simulink model "MPCtest"  (R2016a)
settings: Solver=ode45  StartTime=0.0  StopTime=3600  RelTol=1e-3
StartFcn:
  | % clear all
  | load('mpc');
undefined symbols (not defined in the file or in its folder): model_arx, model_bj, model_oe, model_tf
libraries: slident x5, mpclib x1, realtime_pacer_lib x1
settings Model: Creator=johnh  LastModifiedBy=tiago
settings DataIOCC: SaveFormat=StructureWithTime
settings OptimizationCC: BlockReduction=off  DefaultParameterBehavior=Inlined  BufferReuse=off
settings HardwareCC: ProdWordSize=32  ProdHWDeviceType=Specified
settings ConfigComp: CovModelRefEnable=Off

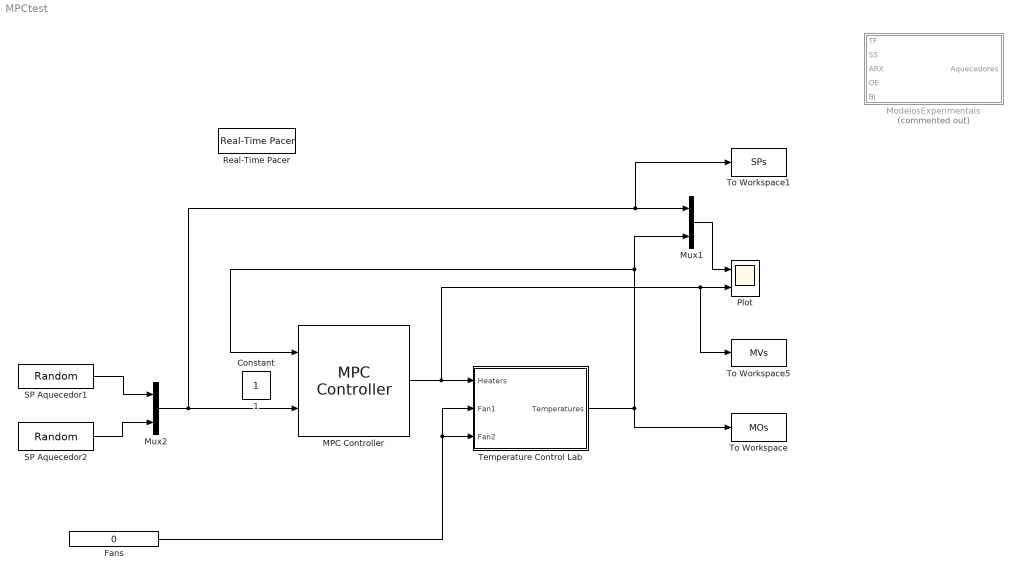
== system MPCtest ==
  Fans : Constant  Value=0
  MPC Controller : mpclib/MPC Controller  SCDEnableBlockLinearizationSpecification=on  mpcobj=mpc_teoricSS_MOWeights10  is_multiple=0  enable_value=0  return_u0=off  ref_from_ws=off  ref_signal_name=[]  ref_preview=off  md_from_ws=off  md_signal_name=[]  md_preview=off  from_project=off  project_file=MPCtask.mat  md_inport=off  mv_inport=off  cost_outport=off  return_sequence=off  return_qpstatus=off  return_state=off  state_inport=off  lims_inport=off  ywt_inport=off  is_designfromscratch=0  uwt_inport=off  duwt_inport=off  rhoeps_inport=off  uref_inport=off  n_ts=7  n_mv=2  n_md=0  n_ud=0  n_mo=2  n_uo=0  BlockDataType=double  SampleTimeInherited=off  switch_inport=off
  ModelosExperimentais : Subsystem  Commented=on
  Mux1 : Mux  Inputs=2
  Mux2 : Mux  Inputs=2
  Plot : Scope  NumInputPorts=2
  Real-Time Pacer : realtime_pacer_lib/Real-Time Pacer  simTimePerRealTime=1
  SP Aquecedor1 : RandomNumber  Mean=50  Variance=25  Seed=90  SampleTime=500
  SP Aquecedor2 : RandomNumber  Mean=50  Variance=25  Seed=91  SampleTime=560
  Temperature Control Lab : Subsystem
      mask Display: image('tclab.png');
  To Workspace : ToWorkspace  VariableName=MOs  SaveFormat=Timeseries  SampleTime=-1
  To Workspace1 : ToWorkspace  VariableName=SPs  SaveFormat=Timeseries  SampleTime=-1
  To Workspace5 : ToWorkspace  VariableName=MVs  SaveFormat=Timeseries  SampleTime=-1
  1 : Constant  IOType=siggen
  Constant : Constant  IOType=siggen
  wires:
  SP Aquecedor1/1 -> Mux2/1
  SP Aquecedor2/1 -> Mux2/2
  Mux2/1 -> Mux1/1, To Workspace1/1, MPC Controller/2
  MPC Controller/1 -> To Workspace5/1, Plot/2, Temperature Control Lab/1(Heaters)
  Fans/1 -> Temperature Control Lab/3(Fan2), Temperature Control Lab/2(Fan1)
  Mux1/1 -> Plot/1
  Temperature Control Lab/1(Temperatures) -> To Workspace/1, Mux1/2, MPC Controller/1

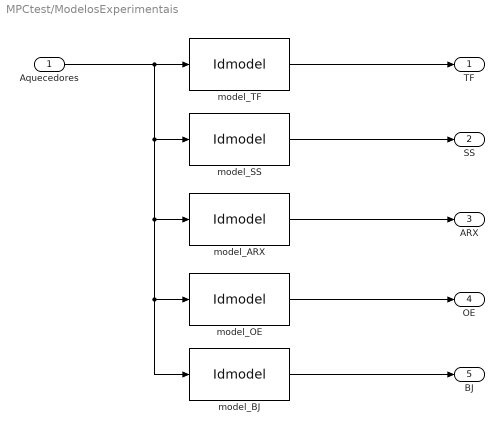
== system MPCtest/ModelosExperimentais ==
  Aquecedores : Inport
  model_ARX : slident/Models/Idmodel  sys=model_arx.model{1,1}  IC=0  noi=on  seed=[]
  model_BJ : slident/Models/Idmodel  sys=model_bj.model{1,1}  IC=0  noi=on  seed=[]
  model_OE : slident/Models/Idmodel  sys=model_oe.model{1,1}  IC=0  noi=on  seed=[]
  model_SS : slident/Models/Idmodel  sys=model_ss  IC=0  noi=on  seed=[]
  model_TF : slident/Models/Idmodel  sys=model_tf.model{1,1}  IC=0  noi=on  seed=[]
  TF : Outport
  SS : Outport  Port=2
  ARX : Outport  Port=3
  OE : Outport  Port=4
  BJ : Outport  Port=5
  wires:
  Aquecedores/1 -> model_BJ/1, model_OE/1, model_ARX/1, model_SS/1, model_TF/1
  model_TF/1 -> TF/1
  model_SS/1 -> SS/1
  model_ARX/1 -> ARX/1
  model_OE/1 -> OE/1
  model_BJ/1 -> BJ/1

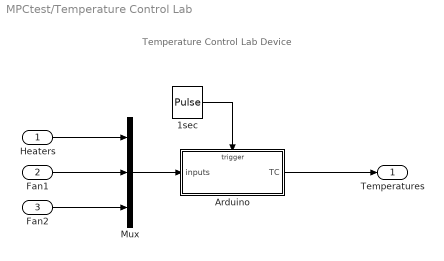
== system MPCtest/Temperature Control Lab ==
  note: Temperature Control Lab Device
  Heaters : Inport  PortDimensions=2
  Fan1 : Inport  Port=2  PortDimensions=1
  Fan2 : Inport  Port=3  PortDimensions=1
  1sec : DiscretePulseGenerator  PulseType=Time based  Period=0.5  PulseWidth=50
  Arduino : Subsystem  TreatAsAtomicUnit=on
  Mux : Mux  Inputs=3
  Temperatures : Outport
  wires:
  1sec/1 -> Arduino/Trigger
  Arduino/1(TC) -> Temperatures/1
  Mux/1 -> Arduino/1(inputs)
  Heaters/1 -> Mux/1
  Fan2/1 -> Mux/3
  Fan1/1 -> Mux/2

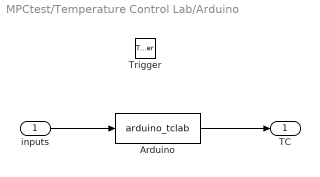
== system MPCtest/Temperature Control Lab/Arduino ==
  inputs : Inport  PortDimensions=4  LatchByDelayingOutsideSignal=on
  Trigger : TriggerPort  VariantControl=Variant
  Arduino : MATLABFcn  MATLABFcn=arduino_tclab
  TC : Outport  InitialOutput=[23 23]
  wires:
  inputs/1 -> Arduino/1
  Arduino/1 -> TC/1
